simulink model "Sim_Model"  (R2023b)
settings: Solver=VariableStepAuto  StartTime=0.0  StopTime=5.1  RelTol=1e-3
values from neighbouring files (symbols this model uses):
  A = 1    [save_constellation_img_from_MATLAB.m]    (also in savedata_imbalance.m)
  fc = 2000    [save_constellation_img_from_MATLAB.m]    (also in savedata_imbalance.m)
  ini_seed1 = randi([0,10000])    [save_constellation_img_from_MATLAB.m]    (also in savedata_imbalance.m)
  ini_seed2 = randi([0,10000])    [save_constellation_img_from_MATLAB.m]    (also in savedata_imbalance.m)
  m_ary = 2    [save_constellation_img_from_MATLAB.m]    (also in savedata_imbalance.m)
  p_offset = p_offset_list(p_offset_counter)    [save_constellation_img_from_MATLAB.m]    (also in savedata_imbalance.m)
  Q_Gain = 1    [save_constellation_img_from_MATLAB.m]    (also in savedata_imbalance.m)
  T_delay = 0    [save_constellation_img_from_MATLAB.m]    (also in savedata_imbalance.m)
libraries: dspsrcs4 x4, commfilt2 x4, commdigbbndam3 x2, commdigbbndpm3 x2, commchan3 x1, commdigbbndapm x1, commrflib2 x1, commrandsrc3 x1
settings Model: Creator="wang  zhiming"  LastModifiedBy=www02
settings OptimizationCC: ReuseModelBlockBuffer=off

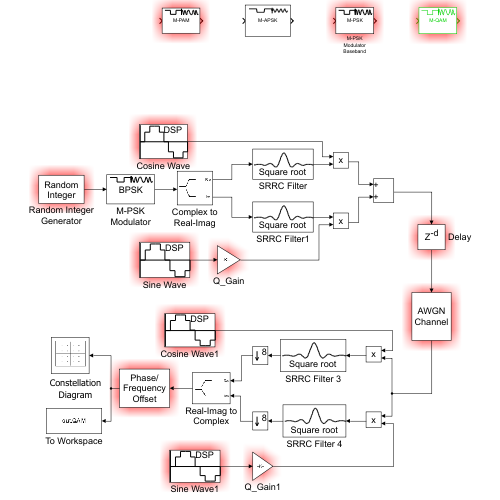
[thumbnail: Simulink's stored preview of the top-level diagram]
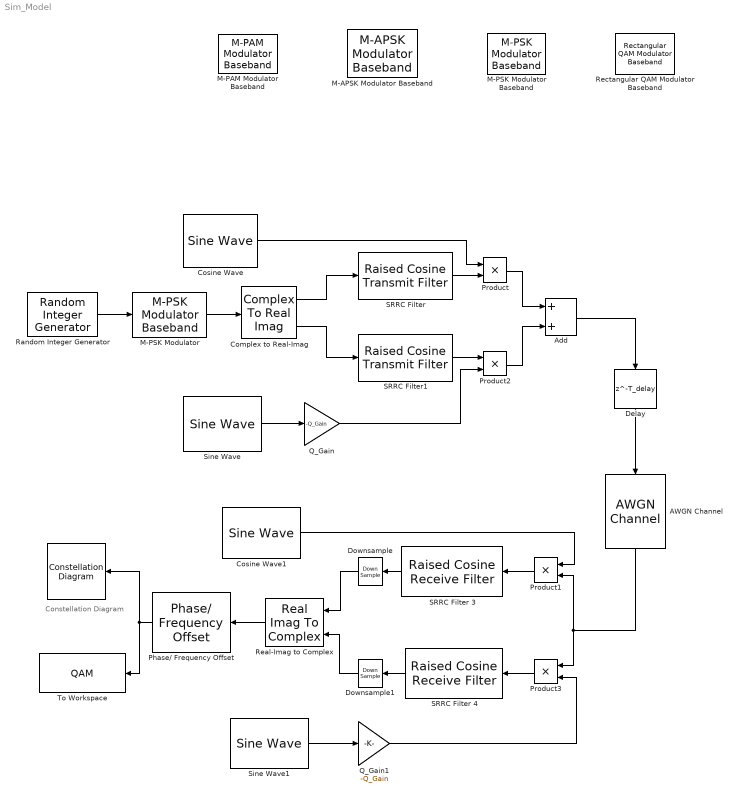
== system Sim_Model ==
  note: Constellation
      | Diagram
  " " : ConstellationDiagram  WindowPosition=[676.000000,166.000000,600.000000,600.000000,]  ScopeFrameLocation=window  SymbolsToDisplaySource=Property  SymbolsToDisplay=1000  XLimits=[-1.46,1.46]  YLimits=[-1.38,1.38]  DefaultConfigurationName=comm.scopes.ConstellationDiagramBlockCfg
  AWGN Channel : commchan3/AWGN Channel  LegacyMode=on  NoiseMethod="Signal to noise ratio  (SNR)"  noiseMode="Signal to noise ratio  (SNR)"  EbNo=10  EsNo=10  SNR=snr_value  BitsPerSymbol=1  SignalPower=1  SamplesPerSymbol=1  SymbolPeriod=1  VarianceSource=Parameter  Variance=1  RandomStream=Global stream  Seed=ini_seed2  SimulateUsing=Code generation
  Add : Sum
  Complex to Real-Imag : ComplexToRealImag
  Cosine Wave : dspsrcs4/Sine Wave  Amplitude=A  Frequency=fc  Phase=pi/2+p_offset  SampleMode=Discrete  OutComplex=Real  CompMethod=Table lookup  TableSize=Speed  SampleTime=1/8000  SamplesPerFrame=1  ResetState=Restart at time zero  OutputFrames=off  dataType=double  wordLen=16  udDataType=sfix(16)  fracBitsMode=Best precision  numFracBits=14  OutDataTypeStr=double  LastOutDataTypeStr=double
  Cosine Wave1 : dspsrcs4/Sine Wave  Amplitude=A  Frequency=fc  Phase=pi/2+p_offset  SampleMode=Discrete  OutComplex=Real  CompMethod=Table lookup  TableSize=Speed  SampleTime=1/8000  SamplesPerFrame=1  ResetState=Restart at time zero  OutputFrames=off  dataType=double  wordLen=16  udDataType=sfix(16)  fracBitsMode=Best precision  numFracBits=15  OutDataTypeStr=double  LastOutDataTypeStr=double
  Delay : Delay  DelayLength=T_delay
  Downsample : DownSample  N=8  RateOptions=Allow multirate processing
  Downsample1 : DownSample  N=8  RateOptions=Allow multirate processing
  M-APSK Modulator Baseband : commdigbbndapm/M-APSK Modulator Baseband  ConstPointsCirclewise=[ 4, 12,16,32 ]  Radii=[ 0.5, 1 ,2, 4]  PhaseOffset=[ pi/4, pi/12, pi/16 , pi/32]  SymbolMapping=Auto  CustomSymbolMapping=[ 0, 4, 12, 8, 1, 3, 2, 6, 7, 5, 13, 15, 14, 10, 11, 9 ]  InputType=Integer  OutputDataType=double  SimulateUsing=Code generation
  M-PAM Modulator Baseband : commdigbbndam3/M-PAM Modulator Baseband  M=m_ary  InType=Integer  Enc=Gray  PowType=Min. distance between symbols  MinDist=2  AvgPow=1  PeakPow=1  outDtype=double  outWordLen=16  outUDDataType=sfix(16)  outFracLenMode=Best precision  outFracLen=15  outDataTypeStr=double  outLastDataTypeStr=double
  "M-PSK Modulator " : commdigbbndpm3/M-PSK Modulator Baseband  M=2  InType=Integer  Enc=Gray  Mapping=[0:7]  Ph=0  outDtype=double  outWordLen=16  outUDDataType=sfix(16)  outFracLenMode=Best precision  outFracLen=15  outDataTypeStr=double  outLastDataTypeStr=double
      settings: LibrarySourceBlock=|
      | commhdldigbbndpm/M-PSK
      | Modulator
      | Baseband
  M-PSK Modulator Baseband : commdigbbndpm3/M-PSK Modulator Baseband  M=m_ary  InType=Integer  Enc=Gray  Mapping=[0:7]  Ph=pi/m_ary  outDtype=double  outWordLen=16  outUDDataType=sfix(16)  outFracLenMode=Best precision  outFracLen=15  outDataTypeStr=double  outLastDataTypeStr=double
      settings: LibrarySourceBlock=|
      | commhdldigbbndpm/M-PSK
      | Modulator
      | Baseband
  Phase/ Frequency Offset : commrflib2/Phase// Frequency Offset  phaseOffset=img_p_offset  freqPort=off  freqOffset=fc_offset
  Product{,1..3} (4 alike) : Product
  Q_Gain : Gain  Gain=-Q_Gain
  Q_Gain1 : Gain  Gain=-Q_Gain
  Random Integer Generator : commrandsrc3/Random Integer Generator  SetSize=m_ary  SeedSource=Parameter  Seed=ini_seed1  SampleTime=1e-3  SamplesPerFrame=1  OutputDataType=uint8  SimulateUsing=Interpreted execution
  Real-Imag to Complex : RealImagToComplex
  Rectangular QAM Modulator Baseband : commdigbbndam3/Rectangular QAM Modulator Baseband  M=m_ary  InType=Integer  Enc=Gray  Mapping=[0:15]  PowType=Min. distance between symbols  MinDist=2  AvgPow=1  PeakPow=1  Ph=0  outDtype=double  outWordLen=16  outUDDataType=sfix(16)  outFracLenMode=Best precision  outFracLen=15  outDataTypeStr=double  outLastDataTypeStr=double
  SRRC Filter : commfilt2/Raised Cosine Transmit Filter  filtType=Square root  R=0.2  filtSpan=10  N=8  filterGain=1  RateOptions=Allow multirate processing  framing=Mute  checkCoeff=off  variableName=rcTxFilt  checkGain=Normalized  sampMode=Mute  saveAsFlag=0  currentFiltSpan=10  D=5  launchFVT=on  roundingMode=Floor  overflowMode=off  coeffDataTypeStr=Inherit: Same word length as input  coeffMin=[]  coeffMax=[]  coeffLastDataTypeStr=Inherit: Same word length as input  outputDataTypeStr=Inherit: Same as accumulator  outputMin=[]  outputMax=[]  outputLastDataTypeStr=Inherit: Same as accumulator
      settings: LibrarySourceBlock=|
      | commhdlfilt/Raised Cosine
      | Transmit Filter
  SRRC Filter 3 : commfilt2/Raised Cosine Receive Filter  filtType=Square root  R=0.2  filtSpan=10  N=8  downFactor=1  downOffset=0  filterGain=1  RateOptions=Allow multirate processing  framing=Mute  checkCoeff=off  variableName=rcRxFilt  currentFiltSpan=10  D=5  inputOffset=0  sampMode=Mute  saveAsFlag=0  rateMode=Downsampling  checkGain=Normalized  launchFVT=on  roundingMode=Floor  overflowMode=off  coeffDataTypeStr=Inherit: Same word length as input  coeffMin=[]  coeffMax=[]  coeffLastDataTypeStr=Inherit: Same word length as input  accumDataTypeStr=Inherit: Same as product output  accumLastDataTypeStr=Inherit: Same as product output  outputDataTypeStr=Inherit: Same as accumulator  outputMin=[]  outputMax=[]  outputLastDataTypeStr=Inherit: Same as accumulator
      settings: LibrarySourceBlock=|
      | commhdlfilt/Raised Cosine
      | Receive Filter
  SRRC Filter 4 : commfilt2/Raised Cosine Receive Filter  filtType=Square root  R=0.2  filtSpan=10  N=8  downFactor=1  downOffset=0  filterGain=1  RateOptions=Allow multirate processing  framing=Mute  checkCoeff=off  variableName=rcRxFilt1  currentFiltSpan=10  D=5  inputOffset=0  sampMode=Mute  saveAsFlag=0  rateMode=Downsampling  checkGain=Normalized  launchFVT=on  roundingMode=Floor  overflowMode=off  coeffDataTypeStr=Inherit: Same word length as input  coeffMin=[]  coeffMax=[]  coeffLastDataTypeStr=Inherit: Same word length as input  accumDataTypeStr=Inherit: Same as product output  accumLastDataTypeStr=Inherit: Same as product output  outputDataTypeStr=Inherit: Same as accumulator  outputMin=[]  outputMax=[]  outputLastDataTypeStr=Inherit: Same as accumulator
      settings: LibrarySourceBlock=|
      | commhdlfilt/Raised Cosine
      | Receive Filter
  SRRC Filter1 : commfilt2/Raised Cosine Transmit Filter  filtType=Square root  R=0.2  filtSpan=10  N=8  filterGain=1  RateOptions=Allow multirate processing  framing=Mute  checkCoeff=off  variableName=rcTxFilt1  checkGain=Normalized  sampMode=Mute  saveAsFlag=0  currentFiltSpan=10  D=5  launchFVT=on  roundingMode=Floor  overflowMode=off  coeffDataTypeStr=Inherit: Same word length as input  coeffMin=[]  coeffMax=[]  coeffLastDataTypeStr=Inherit: Same word length as input  outputDataTypeStr=Inherit: Same as accumulator  outputMin=[]  outputMax=[]  outputLastDataTypeStr=Inherit: Same as accumulator
      settings: LibrarySourceBlock=|
      | commhdlfilt/Raised Cosine
      | Transmit Filter
  Sine Wave : dspsrcs4/Sine Wave  Amplitude=A  Frequency=fc  Phase=0  SampleMode=Discrete  OutComplex=Real  CompMethod=Table lookup  TableSize=Speed  SampleTime=1/8000  SamplesPerFrame=1  ResetState=Restart at time zero  OutputFrames=off  dataType=double  wordLen=16  udDataType=sfix(16)  fracBitsMode=Best precision  numFracBits=15  OutDataTypeStr=double  LastOutDataTypeStr=double
  Sine Wave1 : dspsrcs4/Sine Wave  Amplitude=A  Frequency=fc  Phase=0  SampleMode=Discrete  OutComplex=Real  CompMethod=Table lookup  TableSize=Speed  SampleTime=1/8000  SamplesPerFrame=1  ResetState=Restart at time zero  OutputFrames=off  dataType=double  wordLen=16  udDataType=sfix(16)  fracBitsMode=Best precision  numFracBits=15  OutDataTypeStr=double  LastOutDataTypeStr=double
  To Workspace : ToWorkspace  VariableName=QAM  SampleTime=-1
      settings: Save2DSignal=2-D array (concatenate along first dimension)
  wires:
  Q_Gain1/1 -> Product3/2
  Cosine Wave1/1 -> Product1/1
  AWGN Channel/1 -> Product1/2, Product3/1
  Cosine Wave/1 -> Product/1
  SRRC Filter/1 -> Product/2
  Q_Gain/1 -> Product2/2
  Product2/1 -> Add/2
  SRRC Filter1/1 -> Product2/1
  Product1/1 -> SRRC Filter 3/1
  Sine Wave1/1 -> Q_Gain1/1
  Sine Wave/1 -> Q_Gain/1
  SRRC Filter 3/1 -> Downsample/1
  SRRC Filter 4/1 -> Downsample1/1
  Downsample1/1 -> Real-Imag to Complex/2
  Real-Imag to Complex/1 -> Phase/ Frequency Offset/1
  Product/1 -> Add/1
  Complex to Real-Imag/2 -> SRRC Filter1/1
  Complex to Real-Imag/1 -> SRRC Filter/1
  Delay/1 -> AWGN Channel/1
  Phase/ Frequency Offset/1 -> " "/1, To Workspace/1
  Product3/1 -> SRRC Filter 4/1
  Random Integer Generator/1 -> "M-PSK Modulator "/1
  "M-PSK Modulator "/1 -> Complex to Real-Imag/1
  Downsample/1 -> Real-Imag to Complex/1
  Add/1 -> Delay/1
